simulink model "VCU_Harness"  (R2025b)
settings: Solver=ode8  StartTime=0.0  StopTime=inf  FixedStep=0.0001  RelTol=1e-3
settings Model: DataDictionary=rev3_data.sldd  Creator=matat  LastModifiedBy=matat
settings DebuggingCC: ParameterPrecisionLossMsg=none
settings RTWCC: GPUComputeCapability=3.5

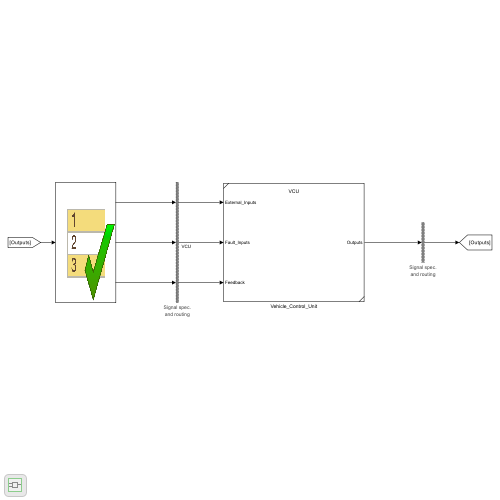
[thumbnail: Simulink's stored preview of the top-level diagram]
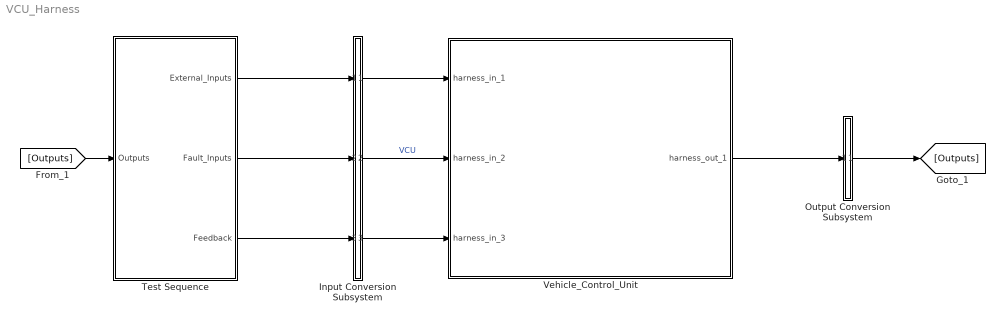
== system VCU_Harness ==
  Input Conversion Subsystem : Subsystem  Tag=__SLT_ICS__  Description=|
      | Signal spec.
      | and routing
      settings: AttributesFormatString=%<Description>
  Output Conversion Subsystem : Subsystem  Tag=__SLT_OCS__  Description=|
      | Signal spec.
      | and routing
      settings: AttributesFormatString=%<Description>
  Test Sequence : Test Sequence  TreatAsAtomicUnit=on
  Vehicle_Control_Unit : Subsystem  Tag=__SL_testing_harness_stub_
  wires:
  Test Sequence/1(External_Inputs) -> Input Conversion Subsystem/1(Inport_1)
  Test Sequence/2(Fault_Inputs) -> Input Conversion Subsystem/2(Inport_2)
  Test Sequence/3(Feedback) -> Input Conversion Subsystem/3(Inport_3)
  [Outputs] -> Test Sequence/1(Outputs)
  Output Conversion Subsystem/1(Outport_1) -> [Outputs]
  Input Conversion Subsystem/1(Outport_1) -> Vehicle_Control_Unit/1(harness_in_1)
  Input Conversion Subsystem/2(Outport_2) -> Vehicle_Control_Unit/2(harness_in_2)  "VCU"
  Input Conversion Subsystem/3(Outport_3) -> Vehicle_Control_Unit/3(harness_in_3)
  Vehicle_Control_Unit/1(harness_out_1) -> Output Conversion Subsystem/1(Inport_1)

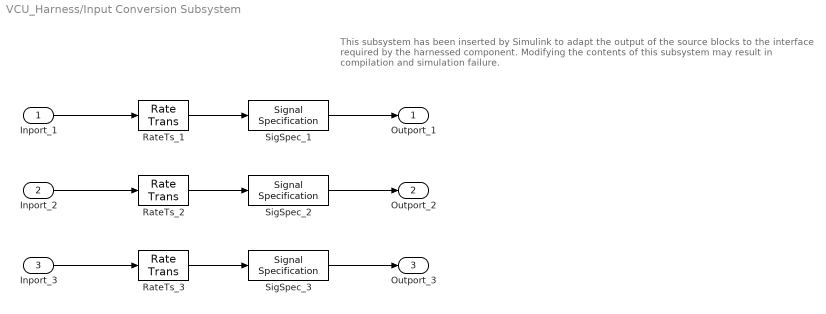
== system VCU_Harness/Input Conversion Subsystem ==
  note: This subsystem has been inserted by Simulink to adapt the output of the source blocks to the interface required by the harnessed component.
      |  Modifying the contents of this subsystem may result in compilation and simulation failure.
  Inport_1 : Inport
  Inport_2 : Inport  Port=2
  Inport_3 : Inport  Port=3
  RateTs_1 : RateTransition  OutPortSampleTime=0.0001
  RateTs_2 : RateTransition  OutPortSampleTime=0.0001
  RateTs_3 : RateTransition  OutPortSampleTime=0.0001
  SigSpec_1 : SignalSpecification  OutDataTypeStr=Bus: External_Inputs  Dimensions=[1]  SampleTime=0.0001  BusOutputAsStruct=on
  SigSpec_2 : SignalSpecification  OutDataTypeStr=Bus: VCU  Dimensions=[1]  SampleTime=0.0001  BusOutputAsStruct=on
  SigSpec_3 : SignalSpecification  OutDataTypeStr=Bus: Feedback_Input  Dimensions=[1]  SampleTime=0.0001  BusOutputAsStruct=on
  Outport_1 : Outport
  Outport_2 : Outport  Port=2
  Outport_3 : Outport  Port=3
  wires:
  SigSpec_1/1 -> Outport_1/1
  RateTs_1/1 -> SigSpec_1/1
  Inport_1/1 -> RateTs_1/1
  SigSpec_2/1 -> Outport_2/1
  RateTs_2/1 -> SigSpec_2/1
  Inport_2/1 -> RateTs_2/1
  SigSpec_3/1 -> Outport_3/1
  RateTs_3/1 -> SigSpec_3/1
  Inport_3/1 -> RateTs_3/1

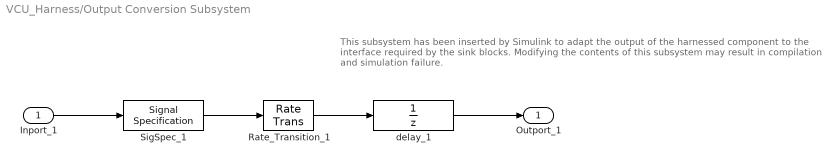
== system VCU_Harness/Output Conversion Subsystem ==
  note: This subsystem has been inserted by Simulink to adapt the output of the harnessed component to the interface required by the sink blocks.
      |  Modifying the contents of this subsystem may result in compilation and simulation failure.
  Inport_1 : Inport
  Rate_Transition_1 : RateTransition  OutPortSampleTimeOpt=Inherit
  SigSpec_1 : SignalSpecification  OutDataTypeStr=Bus: Outputs_VCU  Dimensions=[1]  SampleTime=0.0001  BusOutputAsStruct=on
  delay_1 : UnitDelay  SampleTime=-1
  Outport_1 : Outport
  wires:
  Inport_1/1 -> SigSpec_1/1
  SigSpec_1/1 -> Rate_Transition_1/1
  Rate_Transition_1/1 -> delay_1/1
  delay_1/1 -> Outport_1/1

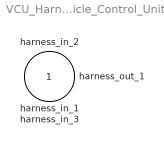
== system VCU_Harness/Vehicle_Control_Unit ==
  harness_in_1 : Inport
  harness_in_2 : Inport  Port=2
  harness_in_3 : Inport  Port=3
  harness_out_1 : Outport

== stateflow chart VCU_Harness/Test Sequence ==
  settings: updateMethod=DISCRETE  sampleTime=0.0001
  state Run
    %% Initialize data outputs.
    External_Inputs.No_HIB.Key_In = false;
    External_Inputs.No_HIB.Estop_In = false;
    External_Inputs.Yes_HIB.HIB_Comparison_Fault = false;
    External_Inputs.Yes_HIB.HIB_Heartbeat = uint32(0);
    External_Inputs.Yes_HIB.Forward_EN = false;
    External_Inputs.Yes_HIB.Start = false;
    External_Inputs.Yes_HIB.Brake = false;
    External_Inputs.Yes_HIB.Throttle = int16(0);
    Fault_Inputs.Override_Ignition = false;
    Fault_Inputs.Ignition = false;
    Fault_Inputs.Override_ESTOP = false;
    Fault_Inputs.ESTOP = false;
    Fault_Inputs.Override_Brake = false;
    Fault_Inputs.Brake = false;
    Fault_Inputs.Override_Forward_EN = false;
    Fault_Inputs.Forward_EN = false;
    Fault_Inputs.Override_Start = false;
    Fault_Inputs.Start = false;
    Fault_Inputs.Override_Throttle = false;
    Fault_Inputs.Throttle = 0;
    Fault_Inputs.Override_HIB_Comparison_Fault = false;
    Fault_Inputs.HIB_Comparison_Fault = false;
    Fault_Inputs.Override_Interlock = false;
    Fault_Inputs.Interlock = false;
    Fault_Inputs.Override_Inverter_Discharge_State = false;
    Fault_Inputs.Inverter_Discharge_State = MC_DC_State.Disabled;
    Fault_Inputs.Override_VSM_State = false;
    Fault_Inputs.VSM_State = MC_VSM_State.Start;
    Fault_Inputs.Override_LVSS_ON = false;
    Fault_Inputs.LVSS_ON = false;
    Fault_Inputs.Override_Contactor_Closed = false;
    Fault_Inputs.Contactor_Closed = false;
    Fault_Inputs.Override_Cell_Temps = false;
    Fault_Inputs.Cell_Temps = 0;
    Fault_Inputs.Override_Cell_Voltages = false;
    Fault_Inputs.Cell_Voltages = 0;
    Fault_Inputs.Override_Isolation_State = false;
    Fault_Inputs.Isolation_State = 0;
    Fault_Inputs.Override_MC_Speed_Out = false;
    Fault_Inputs.MC_Speed_Out = 0;
    Fault_Inputs.Override_Batt_Speed_Out = false;
    Fault_Inputs.Batt_Speed_Out = 0;
    Fault_Inputs.Override_Temperatures = false;
    Fault_Inputs.Temperatures = 0;
    Fault_Inputs.Override_MC_Flow_Rate = false;
    Fault_Inputs.MC_Flow_Rate = 0;
    Fault_Inputs.Override_Batt_Flow_Rate = false;
    Fault_Inputs.Batt_Flow_Rate = 0;
    Fault_Inputs.Override_HIB_ON = false;
    Fault_Inputs.HIB_ON = false;
    Fault_Inputs.Override_HUDL_ON = false;
    Fault_Inputs.HUDL_ON = false;
    Fault_Inputs.Override_TMS_ON = false;
    Fault_Inputs.TMS_ON = false;
    Fault_Inputs.Override_GUB_ON = false;
    Fault_Inputs.GUB_ON = false;
    Fault_Inputs.Override_Acc_ON = false;
    Fault_Inputs.Acc_ON = false;
    Fault_Inputs.Override_Batt_12V_ON = false;
    Fault_Inputs.Batt_12V_ON = false;
    Fault_Inputs.Override_Vicor_Current = false;
    Fault_Inputs.Vicor_Current = 0;
    Fault_Inputs.Override_LVSS_Temps = false;
    Fault_Inputs.LVSS_Temps = 0;
    Fault_Inputs.Override_LVSS_Currents = false;
    Fault_Inputs.LVSS_Currents = 0;
    Fault_Inputs.Override_Heartbeats = false;
    Fault_Inputs.Heartbeats = 0;
    Fault_Inputs.Override_MC_12V0 = false;
    Fault_Inputs.MC_12V0 = false;
    Fault_Inputs.Override_LVSS_EN = false;
    Fault_Inputs.LVSS_EN = false;
    Fault_Inputs.Override_nReset = false;
    Fault_Inputs.nReset = false;
    Fault_Inputs.Override_Self_Test = false;
    Fault_Inputs.Self_Test = 0;
    Fault_Inputs.Override_Watchdog = false;
    Fault_Inputs.Watchdog = false;
    Fault_Inputs.Override_uC_State = false;
    Fault_Inputs.uC_State = UC_State.Preset;
    Fault_Inputs.Override_HB_Feedback = false;
    Fault_Inputs.HB_Feedback = false;
    Fault_Inputs.Override_HM_Fault = false;
    Fault_Inputs.HM_Fault = false;
    Fault_Inputs.Direction_Command = int16(0);
    Fault_Inputs.Override_Direction_Command = false;
    Fault_Inputs.Rolling_Counter = int16(0);
    Fault_Inputs.Override_Rolling_Counter = false;
    Fault_Inputs.Speed_Command = int16(0);
    Fault_Inputs.Override_Speed_Command = false;
    Fault_Inputs.Speed_Mode_Enable = int16(0);
    Fault_Inputs.Override_Speed_Mode_Enable = false;
    Fault_Inputs.Torque_Limit_Command = int16(0);
    Fault_Inputs.Override_Torque_Limit_Command = false;
    Fault_Inputs.LS_Self_Test = false;
    Fault_Inputs.Override_LS_Self_Test = false;
    Fault_Inputs.MC_Self_Test = false;
    Fault_Inputs.Override_MC_Self_Test = false;
    Fault_Inputs.CAN_Self_Test = false;
    Fault_Inputs.Override_CAN_Self_Test = false;
    Fault_Inputs.LVSS_EN_Override = false;
    Fault_Inputs.Override_LVSS_EN_Override = false;
    Fault_Inputs.MC_EN_Override = false;
    Fault_Inputs.Override_MC_EN_Override = false;
    Fault_Inputs.CAN_Override = false;
    Fault_Inputs.Override_CAN_Override = false;
    Feedback_Bus.MC_Feedback.D1_VSM_State = MC_VSM_State.Start;
    Feedback_Bus.MC_Feedback.D4_Inverter_Discharge_State = MC_DC_State.Disabled;
    Feedback_Bus.LVSS_Outputs.HIB_Power = false;
    Feedback_Bus.LVSS_Outputs.HUDL_Power = false;
    Feedback_Bus.LVSS_Outputs.TMS_Power = false;
    Feedback_Bus.LVSS_Outputs.GUB_Power = false;
    Feedback_Bus.LVSS_Outputs.Acc_Power = false;
    Feedback_Bus.LVSS_Outputs.Batt_12V_Power = false;
    Feedback_Bus.LVSS_Feedback.HIB_ON = false;
    Feedback_Bus.LVSS_Feedback.HUDL_ON = false;
    Feedback_Bus.LVSS_Feedback.TMS_ON = false;
    Feedback_Bus.LVSS_Feedback.GUB_ON = false;
    Feedback_Bus.LVSS_Feedback.Acc_ON = false;
    Feedback_Bus.LVSS_Feedback.Batt_12V_ON = false;
    Feedback_Bus.LVSS_Feedback.Vicor_Current = int16(0);
    Feedback_Bus.LVSS_Feedback.LVSS_ON = false;
    Feedback_Bus.LVSS_Feedback.LVSS_Temps = zeros(1,6);
    Feedback_Bus.LVSS_Feedback.LVSS_Currents = zeros(1,6);
    Feedback_Bus.LVSS_Feedback.LVSS_Heartbeat = uint32(0);
    Feedback_Bus.BMS_Feedback.BMS_Heartbeat = uint32(0);
    Feedback_Bus.BMS_Feedback.Cell_Voltages = zeros(1,100);
    Feedback_Bus.BMS_Feedback.Cell_Temps = zeros(1,45);
    Feedback_Bus.BMS_Feedback.Contactor_Closed = false;
    Feedback_Bus.TMS_Feedback.Batt_Flow_Rate = 0;
    Feedback_Bus.TMS_Feedback.MC_Flow_Rate = 0;
    Feedback_Bus.TMS_Feedback.TMS_Heartbeat = uint32(0);
    Feedback_Bus.TMS_Feedback.Temperatures = zeros(1,5);
    Feedback_Bus.TMS_Feedback.Batt_Speed_Out = 0;
    Feedback_Bus.TMS_Feedback.MC_Speed_Out = 0;
    Feedback_Bus.GFDB_Feedback.Isolation_State = 0;
    Feedback_Bus.GFDB_Feedback.GFDB_Heartbeat = uint32(0);
  (default) -> Run
  data: Outputs input Bus: Outputs_VCU size=[1]; External_Inputs output Bus: External_Inputs size=[1]; Fault_Inputs output Bus: VCU size=[1]; Feedback output Bus: Feedback_Input size=[1]
